simulink library "translational_PTO"  (R2024a)
settings: Solver=VariableStepAuto  StartTime=0.0  StopTime=10.0  RelTol=1e-3
undefined symbols (not defined in the file): pistonStrokeLength, pressureIntenseFactor, pto, simu, X, Y, Z
libraries: nesl_utility x24, fl_lib x17, SimscapeFluids_lib x14, sm_lib x5, piston_pump_RO_unit_lib x2, sdl_lib x1, pressure_intensifier_simple x1
(part 2 of 2)

== matlab function translational_PTO/Translational PTO_Wave Glider/MATLAB Function ==
  data: p_in input; qw output
function qw   = RO(p_in)
%S = 4.9087e-4; % membrane area (m2)
P_osm = 2480; % osmotic pressure (kPa)
%Kw = 2.5e-7; % membrane permeability coefficient (m2/s*kPa)
%d = 1; % membrane thickness
%intense_factor = 1; % hydraulic intensifier factor
min_feed_pressure = 5.58e6; % minimum feed pressure, Pa
qw = 0;
if p_in >= min_feed_pressure
    qw = (p_in - P_osm*1000)*2.83e-13; % Rate of water flow through membrane (m3/s)
end
qw(qw<0) = 0; % saturation

%qr = qin - qw; % flow rate of reject water

num_RO_units = 1;
qw = qw*num_RO_units;

== matlab function translational_PTO/Translational PTO_Wave Glider/MATLAB Function2 ==
  data: p_in input; qw output
function qw   = RO(p_in)
%S = 4.9087e-4; % membrane area (m2)
P_osm = 2480; % osmotic pressure (kPa)
%Kw = 2.5e-7; % membrane permeability coefficient (m2/s*kPa)
%d = 1; % membrane thickness
%intense_factor = 1; % hydraulic intensifier factor
min_feed_pressure = 5.58e6; % minimum feed pressure, Pa
qw = 0;
if p_in >= min_feed_pressure
    qw = (p_in - P_osm*1000)*2.83e-13; % Rate of water flow through membrane (m3/s)
end
qw(qw<0) = 0; % saturation

%qr = qin - qw; % flow rate of reject water

num_RO_units = 1;
qw = qw*num_RO_units;

== matlab function translational_PTO/Translational PTO_Wave Glider/MATLAB Function1 ==
  data: u input; y output
function y = fcn(u)

if isnan(u)
    y = 0;
else
    y = u;
end
